simulink model "SysID"  (Simulink 10.0)
settings: Solver=ode1  StartTime=0.0  StopTime=8  FixedStep=0.01  MaxStep=0.02  RelTol=1e-3  AbsTol=1e-6
PreLoadFcn:
  | load sysID_xx_data.mat
libraries: mc9s12tool x2, simulink x2
settings Model: Creator=fwornle  LastModifiedBy=bhisma  SimulationMode=external  ExtModeTrigDuration=2500
settings ConfigSet: Description=rtmc9s12target_R2009b
settings SolverCC: AutoScaleAbsTol=off
settings DataIOCC: SignalLoggingSaveFormat=ModelDataLogs  SaveOutput=off  SaveTime=off  SignalLoggingName=sigsOut
settings OptimizationCC: BlockReduction=off  BooleanDataType=off  ExpressionDepthLimit=2147483647  InitFltsAndDblsToZero=on  LifeSpan=1  EfficientTunableParamExpr=on
settings DebuggingCC: SaveWithParameterizedLinksMsg=none  SignalResolutionControl=TryResolveAllWithWarning  MultiTaskDSMMsg=warning  MultiTaskCondExecSysMsg=none  FcnCallInpInsideContextMsg=warning  StateNameClashWarn=warning
settings HardwareCC: ProdBitPerInt=16  ProdBitPerPointer=16  ProdBitPerSizeT=16  ProdBitPerPtrDiffT=16  ProdEndianess=BigEndian  ProdWordSize=16  ProdHWDeviceType=Motorola HC12
settings SFSimCC: MATLABDynamicMemAlloc=off
settings RTWCC: SystemTargetFile=mc9s12.tlc  GenerateMakefile=off  TemplateMakefile=mc9s12.tmf
settings CodeAppCC: IgnoreCustomStorageClasses=off  CustomSymbolStrType=$N$R$M  InternalIdentifier=Classic
settings STFCustomTargetCC: TargetFcnLib=ansi_tfl_tmw.mat  ModelReferenceCompliant=off  IncludeMdlTerminateFcn=off  ERTCustomFileBanners=on  SupportNonInlinedSFcns=off  RemoveResetFunc=on  MATLABClassNameForMDSCustomization=Simulink.SoftwareTarget.ERTCustomization  CPPClassGenCompliant=on  SystemTargetFile=mc9s12.tlc
settings ERTTargetCC: TargetFcnLib=ansi_tfl_tmw.mat  MultiwordLength=2048  ModelReferenceCompliant=off  ParMdlRefBuildCompliant=off  CompOptLevelCompliant=off  ConcurrentExecutionCompliant=off  IncludeMdlTerminateFcn=off  CombineOutputUpdateFcns=off  SupportContinuousTime=on  ModelStepFunctionPrototypeControlCompliant=off  GRTInterface=on  UseToolchainInfoCompliant=off  ExtMode=on  ExtModeMexFile=ext_serial_mc9s12_comm  ExtModeMexArgs=1,2,115200  ERTCustomFileTemplate=mc9s12_file_process.tlc  ConvertIfToSwitch=off  SuppressUnreachableDefaultCases=off
settings CustomProperty: DataType=RTWOptions_EnumType_C__Users_fw__SVN_rtmc9s12-target_trunk_rtmc9s12_CW_R2009b_bin_mc9s12_1mc9s12_TargetBoard  Value=Dragon12Plus
settings EnumStrPairs: String=Dragon12
settings ConfigComp: CovExternalEMLEnable=off

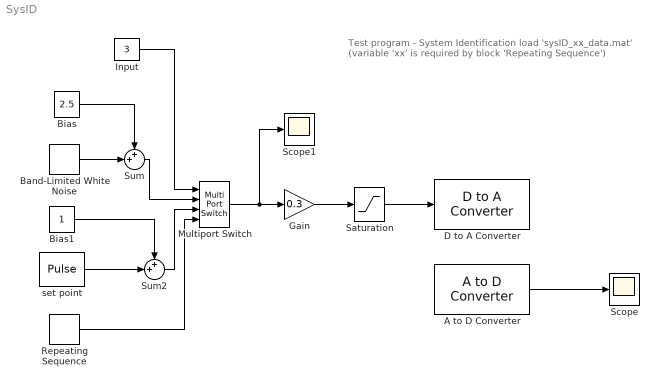
== system SysID ==
  note: Test program - System Identification
      | load 'sysID_xx_data.mat' (variable 'xx'
      | is required by block 'Repeating Sequence')
  A to D Converter : mc9s12tool/A to D Converter  Tag=mcTarget_adc  SystemSampleTime=-1  bank=0  channels=3  use10bits=10 bits  normalize="max. output:  5"  sampletime=0.01
  Band-Limited White Noise : simulink/Sources/Band-Limited White Noise  SystemSampleTime=-1  Cov=[0.05]  Ts=0.1  seed=[23341]
  Bias : Constant  Value=2.5
  Bias1 : Constant
  D to A Converter : mc9s12tool/D to A Converter  Tag=mcTarget_dac  SystemSampleTime=-1  sampletime=0.01  dac_channel=0  Vsat=5
  Gain : Gain  Gain=0.3  SaturateOnIntegerOverflow=on  OutDataTypeStr=Inherit: Same as input  ParamDataTypeStr=Inherit: Same as input
  Input : Constant  Value=3
  Multiport Switch : MultiPortSwitch  SaturateOnIntegerOverflow=on
  Repeating Sequence : simulink/Sources/Repeating Sequence  SystemSampleTime=-1  rep_seq_t=xx.time  rep_seq_y=xx.signals.values
  Saturation : Saturate  UpperLimit=5  LowerLimit=0
  Scope : Scope
  Scope1 : Scope
  Sum : Sum  Inputs=++|  SaturateOnIntegerOverflow=on
  Sum2 : Sum  Inputs=++|  SaturateOnIntegerOverflow=on
  set point : DiscretePulseGenerator  PulseType=Time based  Amplitude=3  PulseWidth=50
  wires:
  Saturation/1 -> D to A Converter/1
  A to D Converter/1 -> Scope/1
  Gain/1 -> Saturation/1
  Bias/1 -> Sum/1
  Band-Limited White Noise/1 -> Sum/2
  Bias1/1 -> Sum2/1
  set point/1 -> Sum2/2
  Sum/1 -> Multiport Switch/2
  Sum2/1 -> Multiport Switch/3
  Input/1 -> Multiport Switch/1
  Repeating Sequence/1 -> Multiport Switch/4
  Multiport Switch/1 -> Gain/1, Scope1/1
